simulink model "sysp4"  (R2023a)
settings: Solver=ode45  StartTime=0.0  StopTime=10.0  MaxStep=1E-3  RelTol=1e-3
settings Model: Creator=Ariel  LastModifiedBy=cesar
settings SolverCC: MaxConsecutiveZCs=10
settings DataIOCC: ReturnWorkspaceOutputs=off  TimeSaveName=t
settings DebuggingCC: AlgebraicLoopMsg=none  ArtificialAlgebraicLoopMsg=none  MaxConsecutiveZCsMsg=none  ModelReferenceExtraNoncontSigs=none  OperatingPointInterfaceChecksumMismatchMsg=none

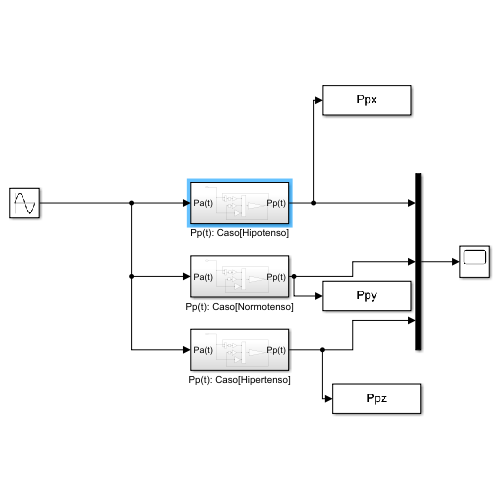
[thumbnail: Simulink's stored preview of the top-level diagram]
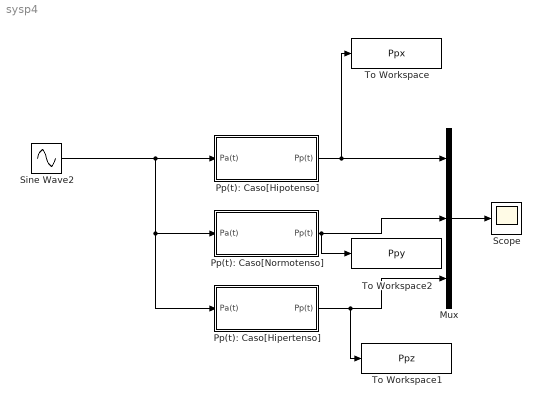
== system sysp4 ==
  Mux : Mux  Inputs=3
  Pp(t): Caso[Hipertenso] : Subsystem
  Pp(t): Caso[Hipotenso] : Subsystem
  Pp(t): Caso[Normotenso] : Subsystem
  Scope : Scope
  Sine Wave2 : Sin  Frequency=(2*pi*95/60)  SampleTime=0
  To Workspace : ToWorkspace  VariableName=Ppx  SaveFormat=Timeseries  SampleTime=-1
  To Workspace1 : ToWorkspace  VariableName=Ppz  SaveFormat=Timeseries  SampleTime=-1
  To Workspace2 : ToWorkspace  VariableName=Ppy  SaveFormat=Timeseries  SampleTime=-1
  wires:
  Mux/1 -> Scope/1
  Pp(t): Caso[Hipotenso]/1(Pp(t)) -> To Workspace/1, Mux/1
  Sine Wave2/1 -> Pp(t): Caso[Normotenso]/1(Pa(t)), Pp(t): Caso[Hipertenso]/1(Pa(t)), Pp(t): Caso[Hipotenso]/1(Pa(t))
  Pp(t): Caso[Normotenso]/1(Pp(t)) -> To Workspace2/1, Mux/2
  Pp(t): Caso[Hipertenso]/1(Pp(t)) -> To Workspace1/1, Mux/3

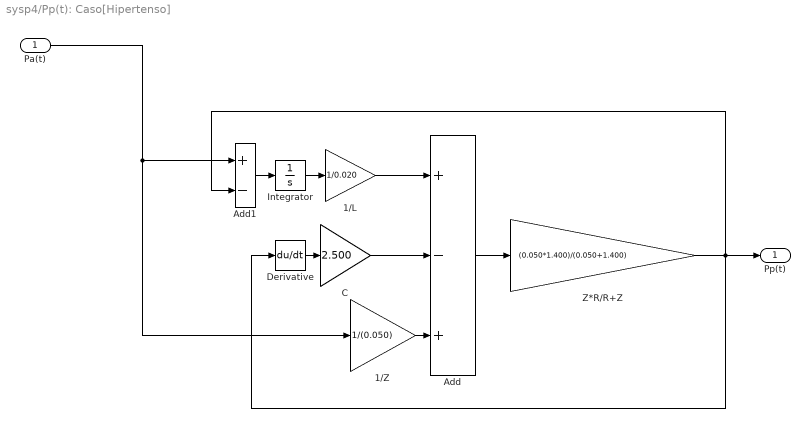
== system sysp4/Pp(t): Caso[Hipertenso] ==
  Pa(t) : Inport
  1/L : Gain  Gain=1/0.020
  1/Z : Gain  Gain=1/(0.050)
  Add : Sum  Inputs=+-+
  Add1 : Sum  Inputs=+-
  C : Gain  Gain=2.500
  Derivative : Derivative
  Integrator : Integrator
  Z*R/R+Z : Gain  Gain=(0.050*1.400)/(0.050+1.400)
  Pp(t) : Outport
  wires:
  Pa(t)/1 -> 1/Z/1, Add1/1
  1/L/1 -> Add/1
  Add/1 -> Z*R/R+Z/1
  Z*R/R+Z/1 -> Derivative/1, Pp(t)/1, Add1/2
  C/1 -> Add/2
  1/Z/1 -> Add/3
  Derivative/1 -> C/1
  Add1/1 -> Integrator/1
  Integrator/1 -> 1/L/1

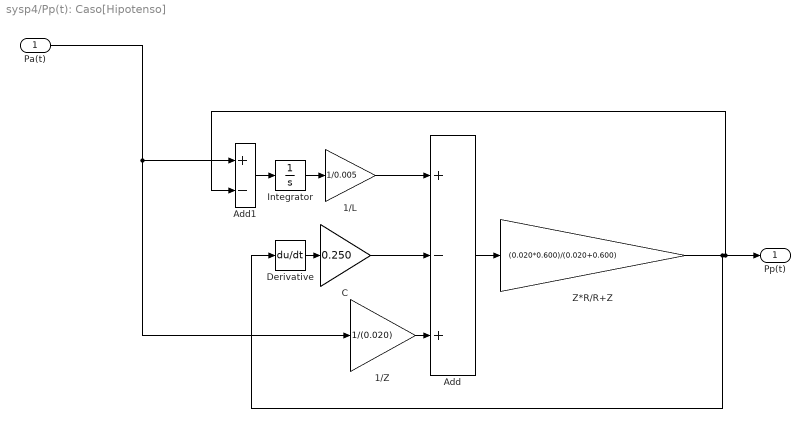
== system sysp4/Pp(t): Caso[Hipotenso] ==
  Pa(t) : Inport
  1/L : Gain  Gain=1/0.005
  1/Z : Gain  Gain=1/(0.020)
  Add : Sum  Inputs=+-+
  Add1 : Sum  Inputs=+-
  C : Gain  Gain=0.250
  Derivative : Derivative
  Integrator : Integrator
  Z*R/R+Z : Gain  Gain=(0.020*0.600)/(0.020+0.600)
  Pp(t) : Outport
  wires:
  Pa(t)/1 -> 1/Z/1, Add1/1
  1/L/1 -> Add/1
  Add/1 -> Z*R/R+Z/1
  Z*R/R+Z/1 -> Derivative/1, Add1/2, Pp(t)/1
  C/1 -> Add/2
  1/Z/1 -> Add/3
  Derivative/1 -> C/1
  Add1/1 -> Integrator/1
  Integrator/1 -> 1/L/1

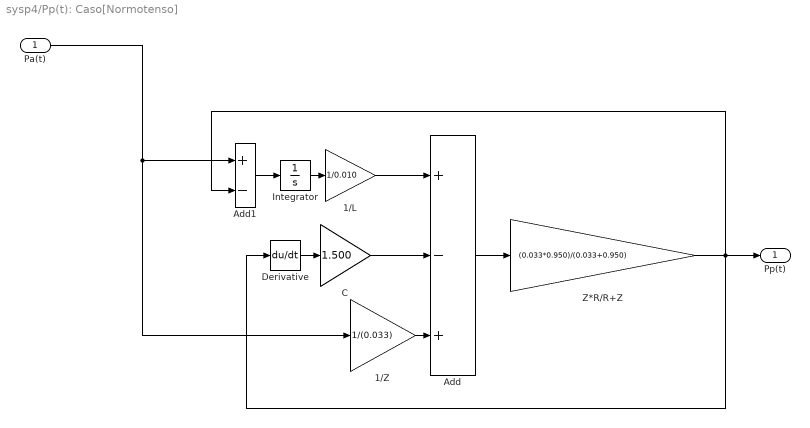
== system sysp4/Pp(t): Caso[Normotenso] ==
  Pa(t) : Inport
  1/L : Gain  Gain=1/0.010
  1/Z : Gain  Gain=1/(0.033)
  Add : Sum  Inputs=+-+
  Add1 : Sum  Inputs=+-
  C : Gain  Gain=1.500
  Derivative : Derivative
  Integrator : Integrator
  Z*R/R+Z : Gain  Gain=(0.033*0.950)/(0.033+0.950)
  Pp(t) : Outport
  wires:
  Pa(t)/1 -> 1/Z/1, Add1/1
  1/L/1 -> Add/1
  Add/1 -> Z*R/R+Z/1
  Z*R/R+Z/1 -> Derivative/1, Pp(t)/1, Add1/2
  C/1 -> Add/2
  1/Z/1 -> Add/3
  Add1/1 -> Integrator/1
  Integrator/1 -> 1/L/1
  Derivative/1 -> C/1
